simulink model "fusionS_22a"  (R2022b)
settings: Solver=VariableStepAuto  StartTime=0.0  StopTime=10.0  RelTol=1e-3
values from neighbouring files (symbols this model uses):
  covA = 800    [fusion_parameters.m]
  covG = 0.0001    [fusion_parameters.m]
  covM = 80    [fusion_parameters.m]
  covP = 34    [fusion_parameters.m]
  covV = 0.0464    [fusion_parameters.m]
  initstate = zeros(28,1)    [fusion_parameters.m]
undefined symbols (not defined in the file or in its folder): acceleration, angularVelocity, MagneticField, position, rateImu, ratioGps, ratioMag, velocity
libraries: sensorgpslib x1, mspsensorlib x1
settings Model: Creator=fullb  LastModifiedBy=Inver

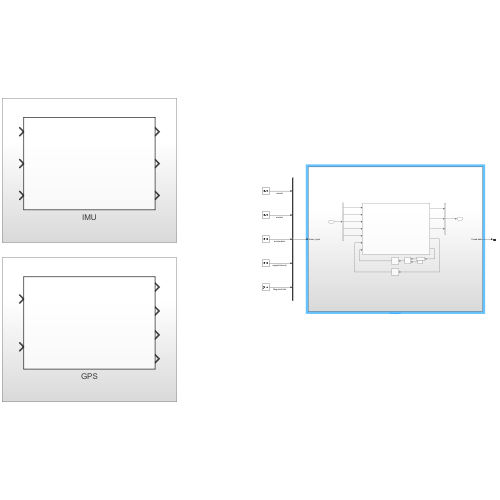
[thumbnail: Simulink's stored preview of the top-level diagram]
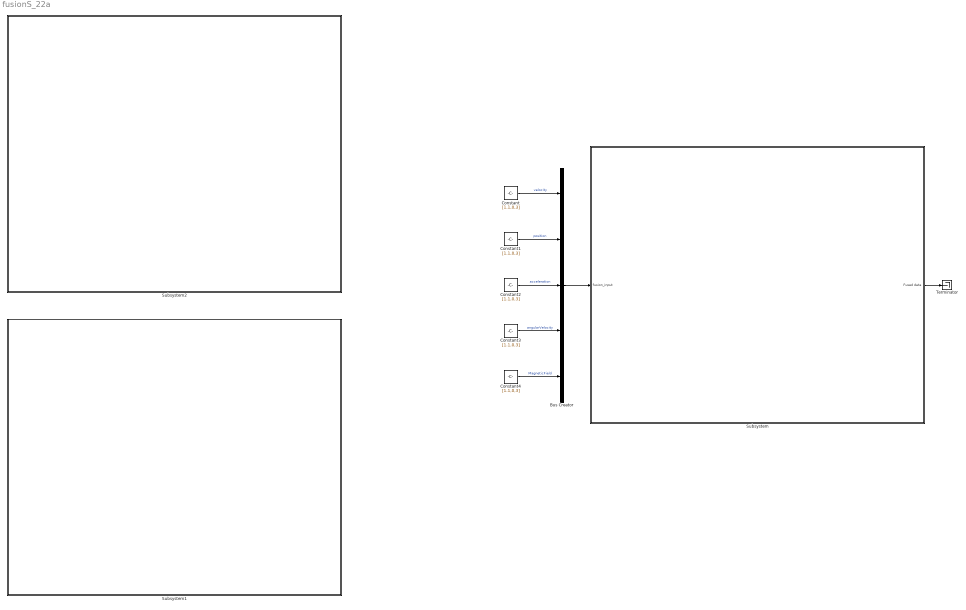
== system fusionS_22a ==
  Bus Creator : BusCreator  Inputs=velocity,position,acceleration,angularVelocity,MagneticField
  Constant{,1..4} (5 alike) : Constant  Value=[1.1,0,3]
  Subsystem : Subsystem
  Subsystem1 : Subsystem
  Subsystem2 : Subsystem
  Terminator : Terminator
  wires:
  Bus Creator/1 -> Subsystem/1(fusion_input)
  Subsystem/1(Fused data) -> Terminator/1
  Constant/1 -> Bus Creator/1  "velocity"
  Constant1/1 -> Bus Creator/2  "position"
  Constant2/1 -> Bus Creator/3  "acceleration"
  Constant3/1 -> Bus Creator/4  "angularVelocity"
  Constant4/1 -> Bus Creator/5  "MagneticField"

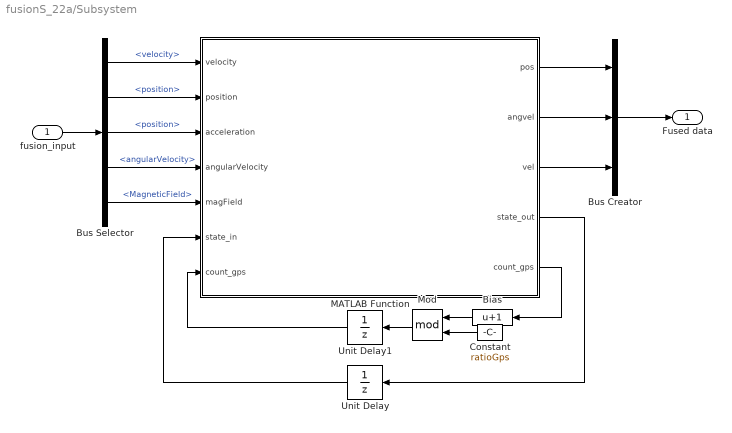
== system fusionS_22a/Subsystem ==
  fusion_input : Inport
  Bias : Bias  Bias=1  SaturateOnIntegerOverflow=off
  Bus Creator : BusCreator  Inputs=3
  Bus Selector : BusSelector  OutputSignals=velocity,position,position,angularVelocity,MagneticField
  Constant : Constant  Value=ratioGps
  MATLAB Function : MATLAB Function  TreatAsAtomicUnit=on
  Mod : Math  Operator=mod
  Unit Delay : UnitDelay  InitialCondition=initstate  SampleTime=t  HasFrameUpgradeWarning=on
  Unit Delay1 : UnitDelay  SampleTime=t  HasFrameUpgradeWarning=on
  Fused data : Outport
  wires:
  Bus Selector/1 -> MATLAB Function/1(velocity)  "<velocity>"
  Bus Selector/4 -> MATLAB Function/4(angularVelocity)  "<angularVelocity>"
  Unit Delay/1 -> MATLAB Function/6(state_in)
  MATLAB Function/5(count_gps) -> Bias/1
  Unit Delay1/1 -> MATLAB Function/7("count_gps ")
  MATLAB Function/4(state_out) -> Unit Delay/1
  Bus Selector/2 -> MATLAB Function/2(position)  "<position>"
  Bus Selector/3 -> MATLAB Function/3(acceleration)  "<position>"
  fusion_input/1 -> Bus Selector/1
  Bus Selector/5 -> MATLAB Function/5(magField)  "<MagneticField>"
  MATLAB Function/1(pos) -> Bus Creator/1
  MATLAB Function/2(angvel) -> Bus Creator/2
  MATLAB Function/3(vel) -> Bus Creator/3
  Bus Creator/1 -> Fused data/1
  Mod/1 -> Unit Delay1/1
  Bias/1 -> Mod/1
  Constant/1 -> Mod/2

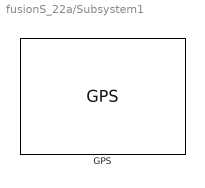
== system fusionS_22a/Subsystem1 ==
  GPS : sensorgpslib/GPS  DispRefFrame=NED  PositionInputFormat=Local  ReferenceLocation=[ 0, 0, 0 ]  HorizontalPositionAccuracy=1.6  VerticalPositionAccuracy=3  VelocityAccuracy=0.1  DecayFactor=0.999  SeedDouble=67  SimulateUsing=Interpreted execution
      settings: LibrarySourceBlock=mspsensorlib/GPS

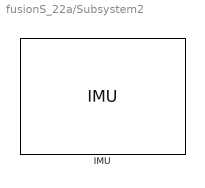
== system fusionS_22a/Subsystem2 ==
  IMU : mspsensorlib/IMU  DispRefFrame=NED  Temperature=25  MagneticFieldNED=[ 27.5550, -2.4169, -16.0849 ]  MagneticFieldENU=[ -2.4169, 27.5550, 16.0849 ]  SeedDouble=67  SimulateUsing=Interpreted execution  AccelParamsMeasurementRange=Inf  AccelParamsResolution=0  AccelParamsConstantBias=[ 0, 0, 0 ]  AccelParamsAxesMisalignment=[ 100, 0, 0; 0, 100, 0; 0, 0, 100 ]  AccelParamsNoiseDensity=[ 0, 0, 0 ]  AccelParamsBiasInstability=[ 0, 0, 0 ]  AccelParamsRandomWalk=[ 0, 0, 0 ]  AccelParamsTemperatureBias=[ 0, 0, 0 ]  AccelParamsTemperatureScaleFactor=[ 0, 0, 0 ]  GyroParamsMeasurementRange=Inf  GyroParamsResolution=0  GyroParamsConstantBias=[ 0, 0, 0 ]  GyroParamsAxesMisalignment=[ 100, 0, 0; 0, 100, 0; 0, 0, 100 ]  GyroParamsAccelerationBias=[ 0, 0, 0 ]  GyroParamsNoiseDensity=[ 0, 0, 0 ]  GyroParamsBiasInstability=[ 0, 0, 0 ]  GyroParamsRandomWalk=[ 0, 0, 0 ]  GyroParamsTemperatureBias=[ 0, 0, 0 ]  GyroParamsTemperatureScaleFactor=[ 0, 0, 0 ]  MagParamsMeasurementRange=Inf  MagParamsResolution=0  MagParamsConstantBias=[ 0, 0, 0 ]  MagParamsAxesMisalignment=[ 100, 0, 0; 0, 100, 0; 0, 0, 100 ]  MagParamsNoiseDensity=[ 0, 0, 0 ]  MagParamsBiasInstability=[ 0, 0, 0 ]  MagParamsRandomWalk=[ 0, 0, 0 ]  MagParamsTemperatureBias=[ 0, 0, 0 ]  MagParamsTemperatureScaleFactor=[ 0, 0, 0 ]

== matlab function fusionS_22a/Subsystem/MATLAB Function ==
  data: pos output; angvel output size=[1,3]; velocity input size=[1,3]; vel output size=[1,3]; state_out output; position input size=[1,3]; acceleration input size=[1,3]; angularVelocity input size=[1,3]; magField input size=[1,3]; state_in input; count_gps input; count_gps output; covG parameter; covA parameter; covM parameter; covP parameter; covV parameter; ratioGps parameter; ratioMag parameter; rateImu parameter
function [pos,angvel,vel, state_out, count_gps] = fusion(velocity, position ,acceleration,angularVelocity, magField,state_in,count_gps, covG, covA, covM, covP, covV, ratioGps, ratioMag, rateImu) 

%creating the filter and loading previous state 
filter.predict((1/rateImu));

%the actual fusion
fuseaccel(filter,acceleration,covA);
fusegyro(filter,angularVelocity,covG);
fusemag(filter, magField,covM);

if ~count_gps
    fusegps(filter,position,covP,velocity,covV);
end
[pos,angvel1,vel] = pose(filter);

angvel = euler(angvel1,"ZYX","Frame");

% update filter state
state_out = filter.State;

end
